simulink model "truck2"  (Simulink 7.3)
settings: Solver=ode45  StartTime=0.0  StopTime=10.0  RelTol=1e-3
settings Model: Creator=Admin  LastModifiedBy=Admin

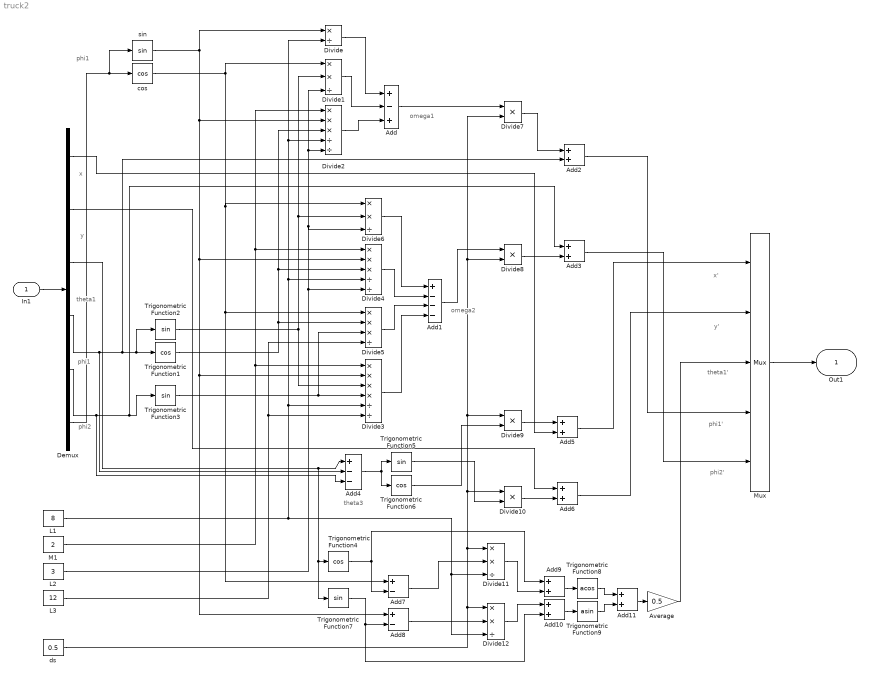
== system truck2 ==
  note: phi1
  note: theta1
  note: y
  note: x
  note: phi2
  note: omega1
  note: omega2
  note: theta3
  note: x'
  note: y'
  note: theta1'
  note: phi1'
  note: phi2'
  note: phi1
  In1 : Inport  OutDataType=fixdt(1, 16)  OutScaling=2^0
  Add : Sum  Inputs=+-+  OutDataType=fixdt(1, 16)  OutScaling=2^-10
  Add1 : Sum  Inputs=+---  OutDataType=fixdt(1, 16)  OutScaling=2^-10
  Add{2..3,5..6,9..11} (7 alike) : Sum  OutDataType=fixdt(1, 16)  OutScaling=2^-10
  Add4 : Sum  Inputs=+--  OutDataType=fixdt(1, 16)  OutScaling=2^-10
  Add7 : Sum  Inputs=+-  OutDataType=fixdt(1, 16)  OutScaling=2^-10
  Add8 : Sum  Inputs=+-  OutDataType=fixdt(1, 16)  OutScaling=2^-10
  Average : Gain  Gain=0.5  ParameterDataType=fixdt(1, 16)  ParameterScaling=2^0  OutDataType=fixdt(1, 16)  OutScaling=2^0
  Demux : Demux  Outputs=6
  Divide : Product  Inputs=*/  OutDataType=fixdt(1, 16)  OutScaling=2^-10
  Divide{1,6,11..12} (4 alike) : Product  Inputs=**/  OutDataType=fixdt(1, 16)  OutScaling=2^-10
  Divide{7..10} (4 alike) : Product  Inputs=**  OutDataType=fixdt(1, 16)  OutScaling=2^-10
  Divide2 : Product  Inputs=***//  OutDataType=fixdt(1, 16)  OutScaling=2^-10
  Divide3 : Product  Inputs=****//  OutDataType=fixdt(1, 16)  OutScaling=2^-10
  Divide4 : Product  Inputs=***//  OutDataType=fixdt(1, 16)  OutScaling=2^-10
  Divide5 : Product  Inputs=***/  OutDataType=fixdt(1, 16)  OutScaling=2^-10
  L1 : Constant  Value=8  OutDataType=fixdt(1, 16)  OutScaling=2^0
  L2 : Constant  Value=3  OutDataType=fixdt(1, 16)  OutScaling=2^0
  L3 : Constant  Value=12  OutDataType=fixdt(1, 16)  OutScaling=2^0
  M1 : Constant  Value=2  OutDataType=fixdt(1, 16)  OutScaling=2^0
  Mux : Mux  Inputs=5
  Trigonometric Function1 : Trigonometry  Operator=cos
  Trigonometric Function{2..3,5,7} (4 alike) : Trigonometry
  Trigonometric Function4 : Trigonometry  Operator=cos
  Trigonometric Function6 : Trigonometry  Operator=cos
  Trigonometric Function8 : Trigonometry  Operator=acos
  Trigonometric Function9 : Trigonometry  Operator=asin
  cos : Trigonometry  Operator=cos
  ds : Constant  Value=0.5  OutDataType=fixdt(1, 16)  OutScaling=2^0
  sin : Trigonometry
  Out1 : Outport  OutDataType=fixdt(1, 16)  OutScaling=2^0
  wires:
  In1/1 -> Demux/1
  sin/1 -> Divide2/2, Divide4/2, Divide3/2, Add8/1, Divide/1
  L1/1 -> Divide2/4, Divide/2, Divide4/4, Divide3/5, Divide11/3, Divide12/3
  L2/1 -> Divide6/3, Divide1/3, Divide2/5, Divide4/5
  cos/1 -> Divide1/1, Divide6/1, Divide5/1, Add7/1
  Demux/4 -> Trigonometric Function2/1, Trigonometric Function1/1, Add2/2, Add4/2
  Trigonometric Function1/1 -> Divide2/3, Divide4/3, Divide5/2
  M1/1 -> Divide2/1, Divide4/1, Divide3/1
  Divide/1 -> Add/1
  Divide1/1 -> Add/2
  Divide2/1 -> Add/3
  Trigonometric Function2/1 -> Divide1/2, Divide6/2, Divide3/3
  Demux/5 -> Add3/1, Trigonometric Function3/1, Add4/3
  Trigonometric Function3/1 -> Divide5/3, Divide3/4
  L3/1 -> Divide5/4, Divide3/6
  Divide6/1 -> Add1/1
  Divide4/1 -> Add1/2
  Divide5/1 -> Add1/3
  Divide3/1 -> Add1/4
  ds/1 -> Divide8/2, Divide7/2, Divide9/1, Divide10/1, Divide11/1, Divide12/1
  Add/1 -> Divide7/1
  Divide7/1 -> Add2/1
  Add1/1 -> Divide8/1
  Divide8/1 -> Add3/2
  Demux/3 -> Add4/1, Trigonometric Function4/1, Trigonometric Function7/1
  Add4/1 -> Trigonometric Function5/1, Trigonometric Function6/1
  Trigonometric Function6/1 -> Divide9/2
  Trigonometric Function5/1 -> Divide10/2
  Divide9/1 -> Add5/1
  Demux/1 -> Add5/2
  Divide10/1 -> Add6/2
  Demux/2 -> Add6/1
  Trigonometric Function4/1 -> Add7/2, Add9/1
  Trigonometric Function7/1 -> Add8/2, Add10/2
  Add7/1 -> Divide11/2
  Add8/1 -> Divide12/2
  Divide11/1 -> Add9/2
  Divide12/1 -> Add10/1
  Add9/1 -> Trigonometric Function8/1
  Add10/1 -> Trigonometric Function9/1
  Trigonometric Function8/1 -> Add11/1
  Trigonometric Function9/1 -> Add11/2
  Add11/1 -> Average/1
  Add2/1 -> Mux/4
  Average/1 -> Mux/3
  Add5/1 -> Mux/1
  Add6/1 -> Mux/2
  Add3/1 -> Mux/5
  Mux/1 -> Out1/1
  Demux/6 -> sin/1, cos/1
